simulink model "buck_converter_closed_loop"  (R2016a)
settings: Solver=ode45  StartTime=0.0  StopTime=2e-3  MaxStep=0.1e-6  RelTol=1e-3
values from neighbouring files (symbols this model uses):
  C = 376e-6    (= 0.000376)    [buck_converter_closed_loop_sim_parameters.m]    (also in buck_converter_open_loop_sim_parameters.m)
  D = 0.42    [buck_converter_closed_loop_sim_parameters.m]    (also in buck_converter_open_loop_sim_parameters.m)
  Gc0 = Gcwcabs/abs((1+i*wc/wz)/(1+i*wc/wp))    [buck_converter_closed_loop_sim_parameters.m]
  L = 4.1e-6    (= 4.1e-06)    [buck_converter_closed_loop_sim_parameters.m]    (also in buck_converter_open_loop_sim_parameters.m)
  Resr = 5e-3    (= 0.005)    [buck_converter_closed_loop_sim_parameters.m]    (also in buck_converter_open_loop_sim_parameters.m)
  RL = 80e-3    (= 0.08)    [buck_converter_closed_loop_sim_parameters.m]    (also in buck_converter_open_loop_sim_parameters.m)
  Rload = 1    [buck_converter_closed_loop_sim_parameters.m]    (also in buck_converter_open_loop_sim_parameters.m)
  Vg = 12    [buck_converter_closed_loop_sim_parameters.m]    (also in buck_converter_open_loop_sim_parameters.m)
  wL = wc/50    (= 1256.63706144)    [buck_converter_closed_loop_sim_parameters.m]
  wp = 2*pi*fp    [buck_converter_closed_loop_sim_parameters.m]
  wz = 2*pi*fz    [buck_converter_closed_loop_sim_parameters.m]
libraries: simulink_extras x1, simulink x1
settings Model: Creator=Gorkem  LastModifiedBy=Gorkem
settings GRTTargetCC: GeneratePreprocessorConditionals=Use local settings

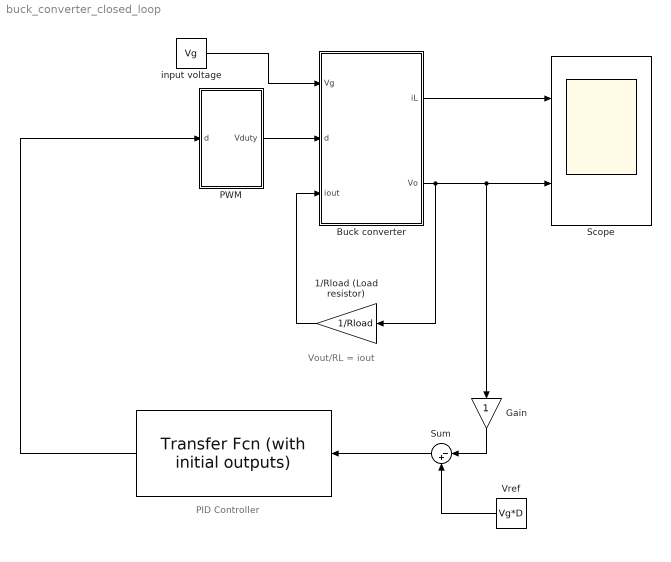
== system buck_converter_closed_loop ==
  note: PID Controller
  note: Vout/RL = iout
  "                                          " : simulink_extras/Additional Linear/Transfer Fcn (with initial outputs)  N="[Gc0/wz  Gc0+wL*(Gc0/wz)  Gc0*wL]"  D="[1/wp  1  0]"  Y0=0.42  U0=0
  1/Rload (Load resistor) : Gain  Gain=1/Rload
  Buck converter : Subsystem
  Gain : Gain
  PWM : Subsystem
  Scope : Scope  NumInputPorts=2
  Sum : Sum  Inputs=|-+
  Vref : Constant  Value=Vg*D
  input voltage : Constant  Value=Vg
  wires:
  input voltage/1 -> Buck converter/1(Vg)
  PWM/1(Vduty) -> Buck converter/2(d)
  1/Rload (Load resistor)/1 -> Buck converter/3(iout)
  Buck converter/1(iL) -> Scope/1
  Buck converter/2(Vo) -> Gain/1, Scope/2, 1/Rload (Load resistor)/1
  Sum/1 -> "                                          "/1
  Gain/1 -> Sum/1
  Vref/1 -> Sum/2
  "                                          "/1 -> PWM/1(d)

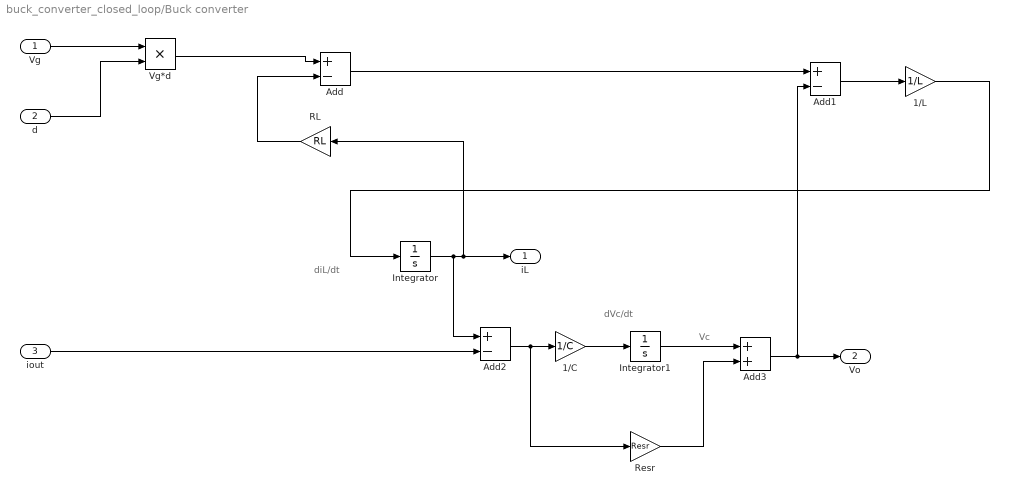
== system buck_converter_closed_loop/Buck converter ==
  note: Vc
  note: dVc/dt
  note: diL/dt
  Vg : Inport
  d : Inport  Port=2
  iout : Inport  Port=3
  1/C : Gain  Gain=1/C
  1/L : Gain  Gain=1/L
  Add : Sum  Inputs=+-
  Add1 : Sum  Inputs=+-
  Add2 : Sum  Inputs=+-
  Add3 : Sum
  Integrator : Integrator
  Integrator1 : Integrator
  RL : Gain  Gain=RL
  Resr : Gain  Gain=Resr
  Vg*d : Product
  iL : Outport
  Vo : Outport  Port=2
  wires:
  1/L/1 -> Integrator/1
  Integrator/1 -> Add2/1, iL/1, RL/1
  Vg/1 -> Vg*d/1
  1/C/1 -> Integrator1/1
  Add2/1 -> Resr/1, 1/C/1
  Vg*d/1 -> Add/1
  Add1/1 -> 1/L/1
  Add3/1 -> Vo/1, Add1/2
  d/1 -> Vg*d/2
  Integrator1/1 -> Add3/1
  Resr/1 -> Add3/2
  RL/1 -> Add/2
  iout/1 -> Add2/2
  Add/1 -> Add1/1

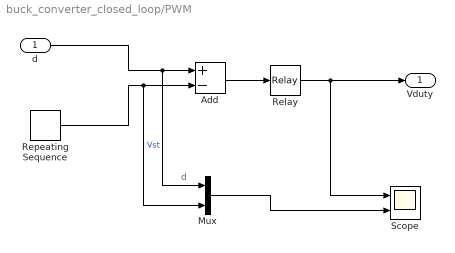
== system buck_converter_closed_loop/PWM ==
  note: d
  d : Inport
  Add : Sum  Inputs=+-
  Mux : Mux  Inputs=2
  Relay : Relay  ZeroCross=off
  Repeating Sequence : simulink/Sources/Repeating Sequence  rep_seq_t=[0 0.001e-5 1e-5]  rep_seq_y=[1 0 1]
  Scope : Scope  NumInputPorts=2
  Vduty : Outport
  wires:
  Relay/1 -> Vduty/1, Scope/1
  Repeating Sequence/1 -> Mux/2, Add/2  "Vst"
  Add/1 -> Relay/1
  Mux/1 -> Scope/2
  d/1 -> Mux/1, Add/1
